simulink model "a_adaptivesInveresFilter"  (Simulink 6.5)
settings: Solver=ode45  StartTime=0.0  StopTime=1000.0  RelTol=1e-3
undefined symbols (not defined in the file): Amplitudengang, Koeffizienten, LMS, RLS
libraries: dspsnks4 x4, dspadpt3 x2, dspspect3 x2, simulink x2
settings Model: Creator=Wirnitzer  LastModifiedBy=Wirnitzer
settings OptimizationCC: BooleanDataType=off
settings DebuggingCC: SolverPrmCheckMsg=none  MultiTaskDSMMsg=warning  MultiTaskCondExecSysMsg=none  StrictBusMsg=None
settings HardwareCC: TargetUnknown=on
settings RTWCC: IncludeERTFirstTime=on
settings GRTTargetCC: ModelReferenceCompliant=off  MatFileLogging=off

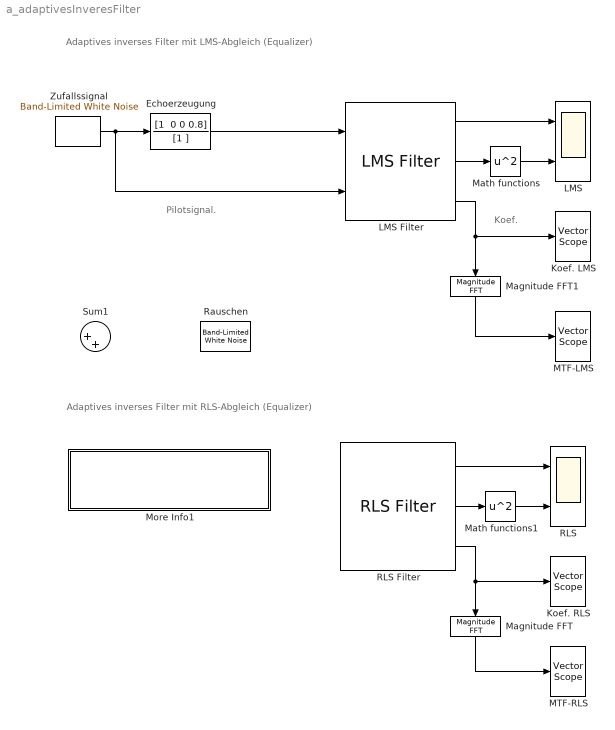
== system a_adaptivesInveresFilter ==
  note: Pilotsignal.
  note: Adaptives inverses  Filter mit RLS-Abgleich
      |  (Equalizer)
  note: Koef.
  note: Adaptives inverses  Filter mit LMS-Abgleich
      | (Equalizer)
  Echoerzeugung : DiscreteFilter  Numerator="[1  0 0 0.8]"  Denominator=[1 ]
  Koef. LMS : dspsnks4/Vector Scope  DialogController=dspdialog.VectorScope  DialogControllerArgs=DataTag0  ScopeProperties=on  Domain=User-defined  HorizSpan=1  DisplayProperties=off  AxisGrid=on  Memory=off  FrameNumber=off  AxisLegend=off  AxisZoom=off  OpenScopeAtSimStart=on  OpenScopeImmediately=off  FigPos=[491 123 450 360]  AxisProperties=off  XUnits=Hertz  XRange=[0...Fs/2]  InheritXIncr=off  XIncr=1  XLabel=Index  YUnits=dB  YLabel=LMS-Koeffizienten  LineProperties=off  LineMarkers=.
      settings: YMin=-0.487309903535585  YMax=0.83885356263275
  Koef. RLS : dspsnks4/Vector Scope  DialogController=dspdialog.VectorScope  DialogControllerArgs=DataTag1  ScopeProperties=on  Domain=User-defined  HorizSpan=1  DisplayProperties=off  AxisGrid=on  Memory=off  FrameNumber=off  AxisLegend=off  AxisZoom=off  OpenScopeAtSimStart=on  OpenScopeImmediately=off  FigPos=[491 123 450 360]  AxisProperties=off  XUnits=Hertz  XRange=[0...Fs/2]  InheritXIncr=off  XIncr=1  XLabel=Index  YUnits=dB  YLabel=RLS-Koeffizienten  LineProperties=off  LineMarkers=.
      settings: YMin=-0.425687335392183  YMax=0.378680117510527
  LMS : Scope  NumInputPorts=2
      settings: AttributesFormatString=test  YMin=-5~-5  YMax=5~5
  LMS Filter : dspadpt3/LMS Filter  DialogController=dspDDGCreate  DialogControllerArgs=DataTag2  Algo=Normalized LMS  L=11  stepflag=Dialog  mu=0.05  leakage=1.0  ic=0  Adapt=off  resetflag=None  weights=on  secondCoeffMode=User-defined  secondCoeffWordLength=2  secondCoeffFracLength=15  accum2Mode=User-defined  accum2FracLength=20  prodOutput2Mode=User-defined  prodOutput2FracLength=20  prodOutput3Mode=User-defined  prodOutput3FracLength=20  prodOutput4Mode=User-defined  prodOutput4FracLength=20  quotientMode=User-defined  quotientFracLength=20  roundingMode=Floor  overflowMode=off  addnparflag=off
  MTF-LMS : dspsnks4/Vector Scope  DialogController=dspdialog.VectorScope  DialogControllerArgs=DataTag3  ScopeProperties=on  Domain=User-defined  HorizSpan=1  DisplayProperties=off  AxisGrid=on  Memory=off  FrameNumber=off  AxisLegend=off  AxisZoom=off  OpenScopeAtSimStart=on  OpenScopeImmediately=off  FigPos=[491 123 450 360]  AxisProperties=off  XUnits=Hertz  XRange=[0...Fs/2]  InheritXIncr=off  XIncr=1  XLabel=Frequenzzahl  YUnits=dB  YLabel=LMS-Amplitudengang  LineProperties=off  LineMarkers=.
      settings: YMin=0.465436697275106  YMax=1.62866851228103
  MTF-RLS : dspsnks4/Vector Scope  DialogController=dspdialog.VectorScope  DialogControllerArgs=DataTag4  ScopeProperties=on  Domain=User-defined  HorizSpan=1  DisplayProperties=off  AxisGrid=on  Memory=off  FrameNumber=off  AxisLegend=off  AxisZoom=off  OpenScopeAtSimStart=on  OpenScopeImmediately=off  FigPos=[491 123 450 360]  AxisProperties=off  XUnits=Hertz  XRange=[0...Fs/2]  InheritXIncr=off  XIncr=1  XLabel=Frequenzzahl  YUnits=dB  YLabel=RLS-Amplitudengang  LineProperties=off  LineMarkers=.
      settings: YMin=0.101196068195768  YMax=1.34327062494384
  Magnitude FFT : dspspect3/Magnitude FFT  Orientation=down  SystemSampleTime=-1  mag_or_magsq=Magnitude  fftLenInherit=off  fftsize=256
  Magnitude FFT1 : dspspect3/Magnitude FFT  Orientation=down  SystemSampleTime=-1  mag_or_magsq=Magnitude  fftLenInherit=off  fftsize=256
  Math functions : Math  Operator=square  SaturateOnIntegerOverflow=on
  Math functions1 : Math  Operator=square  SaturateOnIntegerOverflow=on
  More Info1 : Subsystem
      mask Display: disp(' Aufgaben')
  RLS : Scope  NumInputPorts=2
      settings: TimeRange=400  YMin=-5~13.73684210526316  YMax=5~25.73684210526316
  RLS Filter : dspadpt3/RLS Filter  SystemSampleTime=-1  L=11  lambdaflag=Dialog  lambda=0.999  addnparflag=on  ic=0  delta=0.1  Adapt=off  resetflag=None  weights=on
  Rauschen : simulink/Sources/Band-Limited White Noise  Orientation=up  SystemSampleTime=-1  Cov=0.3  Ts=1  seed=[241]
  Sum1 : Sum  Inputs=|++  SaturateOnIntegerOverflow=on  InputSameDT=on
  Zufallssignal : simulink/Sources/Band-Limited White Noise  SystemSampleTime=-1  Cov=1  Ts=1  seed=[23341]
  wires:
  Math functions/1 -> LMS/2
  LMS Filter/1 -> LMS/1
  LMS Filter/2 -> Math functions/1
  LMS Filter/3 -> Koef. LMS/1, Magnitude FFT1/1
  Zufallssignal/1 -> Echoerzeugung/1, LMS Filter/2
  Math functions1/1 -> RLS/2
  RLS Filter/1 -> RLS/1
  RLS Filter/2 -> Math functions1/1
  RLS Filter/3 -> Koef. RLS/1, Magnitude FFT/1
  Magnitude FFT/1 -> MTF-RLS/1
  Magnitude FFT1/1 -> MTF-LMS/1
  Echoerzeugung/1 -> LMS Filter/1

== system a_adaptivesInveresFilter/More Info1 ==
  note: Adaptives Inverses System (== Entzerrer == Equalizer)
      | ===========================================
      | (c) HSM, B. Wir 7.11 97, 8.8.2012
      |
      |
      | Starten Sie die Simulation mit  SIMULATION, START.
      | Beobachten Sie wie sich die Koeffizienten des Filters langsam einstellen.
      | Durch einen Doppelklick auf das Oszilloskop können Sie die Signale
      | beobachten. Mit der rechten Maustate können Sie AUTOSCALE aktivieren.
      |
      | (i)   Stellen sich die erwarteten Filterkoeffizienten ein?
      |
      | (ii)  Welche Einflüsse haben die Filterordnung und die Schrittweite des LMS auf das Ergebnis?
      |
      | (iii) Addieren Sie Rauschen zum System und untersuchen Sie (i) und (ii).
      |
      | (iv) Welche Vorteile bringt der RLS-Algorithmus?
      |
      | (v)  Entzerren Sie den Übertragungskanal \( G(z) = 1 + 2z^{-1} + z^{-3} \) und beantworten Sie (i)-(iv).
